simulink model "label_traj_calc"  (R2020b)
settings: Solver=FixedStepDiscrete  StartTime=0.0  StopTime=10.0  FixedStep=0.05  RelTol=1e-3
libraries: simulink x1
settings Model: Creator=chaoqun  LastModifiedBy=chaoqun
settings OptimizationCC: DefaultParameterBehavior=Inlined  EnhancedBackFolding=on  PassReuseOutputArgsAs=Individual arguments  ZeroExternalMemoryAtStartup=off  ZeroInternalMemoryAtStartup=off  OptimizeBlockOrder=speed  DifferentSizesBufferReuse=on  OptimizationCustomize=off  EfficientTunableParamExpr=on
settings DebuggingCC: ParameterTunabilityLossMsg=error
settings SFSimCC: MATLABDynamicMemAlloc=off
settings RTWCC: Description=Embedded Coder  SystemTargetFile=ert.tlc  GenCodeOnly=on  TemplateMakefile=ert_default_tmf
settings CodeAppCC: ForceParamTrailComments=on  IgnoreCustomStorageClasses=off  OperatorAnnotations=on  SimulinkDataObjDesc=on  SFDataObjDesc=on  InsertBlockDesc=on
settings ERTTargetCC: TargetLangStandard=C99 (ISO)  InlinedParameterPlacement=NonHierarchical  ERTCustomFileTemplate=example_file_process.tlc

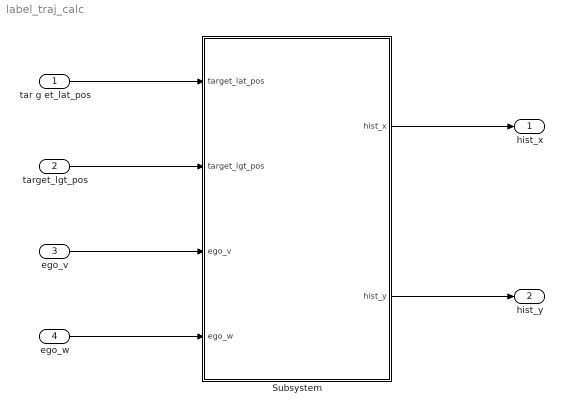
== system label_traj_calc ==
  tar g et_lat_pos : Inport  PortDimensions=100
  target_lgt_pos : Inport  Port=2  PortDimensions=100
  ego_v : Inport  Port=3  PortDimensions=100
  ego_w : Inport  Port=4  PortDimensions=100
  Subsystem : Subsystem
  hist_x : Outport
  hist_y : Outport  Port=2
  wires:
  tar g et_lat_pos/1 -> Subsystem/1(target_lat_pos)
  target_lgt_pos/1 -> Subsystem/2(target_lgt_pos)
  ego_v/1 -> Subsystem/3(ego_v)
  ego_w/1 -> Subsystem/4(ego_w)
  Subsystem/1(hist_x) -> hist_x/1
  Subsystem/2(hist_y) -> hist_y/1

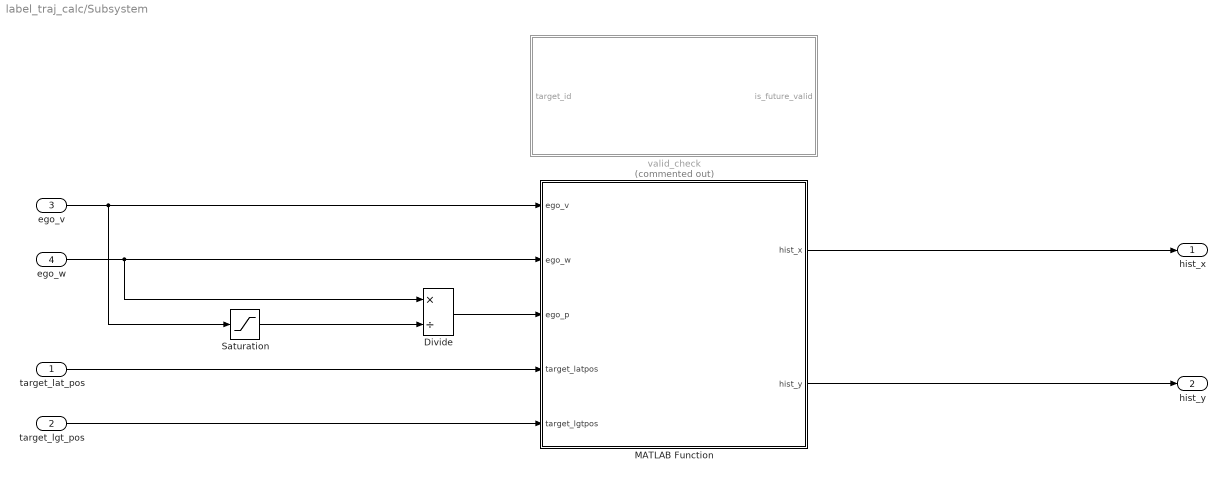
== system label_traj_calc/Subsystem ==
  target_lat_pos : Inport  PortDimensions=100
  target_lgt_pos : Inport  Port=2  PortDimensions=100
  ego_v : Inport  Port=3  PortDimensions=100
  ego_w : Inport  Port=4  PortDimensions=100
  Divide : Product  Inputs=*/
  MATLAB Function : MATLAB Function  TreatAsAtomicUnit=on
  Saturation : Saturate  UpperLimit=100  LowerLimit=1
  valid_check : Subsystem  Commented=on
  hist_x : Outport
  hist_y : Outport  Port=2
  wires:
  ego_w/1 -> MATLAB Function/2(ego_w), Divide/1
  Divide/1 -> MATLAB Function/3(ego_p)
  target_lat_pos/1 -> MATLAB Function/4(target_latpos)
  target_lgt_pos/1 -> MATLAB Function/5(target_lgtpos)
  MATLAB Function/2(hist_y) -> hist_y/1
  Saturation/1 -> Divide/2
  ego_v/1 -> MATLAB Function/1(ego_v), Saturation/1
  MATLAB Function/1(hist_x) -> hist_x/1

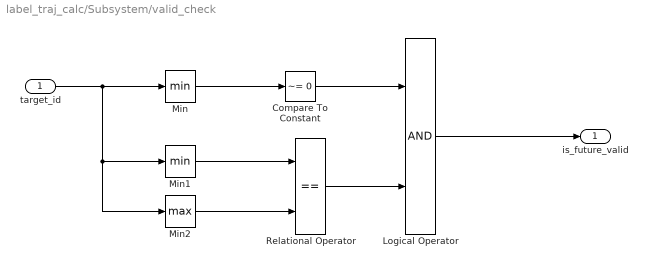
== system label_traj_calc/Subsystem/valid_check ==
  target_id : Inport
  Compare To Constant : simulink/Logic and Bit Operations/Compare To Constant  relop=~=  const=0  OutDataTypeStr=boolean
  Logical Operator : Logic  AllPortsSameDT=off  OutDataTypeStr=boolean
  Min : MinMax
  Min1 : MinMax
  Min2 : MinMax  Function=max
  Relational Operator : RelationalOperator  Operator===  OutDataTypeStr=boolean  RndMeth=Simplest
  is_future_valid : Outport
  wires:
  target_id/1 -> Min2/1, Min1/1, Min/1
  Min/1 -> Compare To Constant/1
  Compare To Constant/1 -> Logical Operator/1
  Relational Operator/1 -> Logical Operator/2
  Min2/1 -> Relational Operator/2
  Min1/1 -> Relational Operator/1
  Logical Operator/1 -> is_future_valid/1

== matlab function label_traj_calc/Subsystem/MATLAB Function ==
  data: ego_v input; ego_w input; ego_p input; target_latpos input; target_lgtpos input; hist_x output; hist_y output
function [hist_x, hist_y] = fcn(ego_v, ego_w, ego_p, target_latpos, target_lgtpos)

    hist_x = zeros(1,100);
    hist_y = zeros(1,100);

    dt = 0.05;


    for i=1:1:100
        psi= ego_w(100-i+1)*dt;

        dX = ego_v(100-i+1)*dt;

        dY = 0.5*ego_p(100-i+1)*dX*dX;


        % assign new target(x,y)
        hist_x(1, 100-i+1) = target_lgtpos(100-i+1);
        hist_y(1, 100-i+1) = target_latpos(100-i+1);


        [hist_x, hist_y] = coords_translate(-1*psi, -1*dX, -1*dY, hist_x, hist_y);


    end


end




function [X_t, Y_t] =  coords_translate(psi, dX, dY, X, Y)
% /*
% Transform Matrix is as following:   Move (dX, dY)m, Then Rotate (Psi) rad
% 
%          [  cos(psi)  sin(psi)  -(dX*cos(psi) + dY*sin(psi)) ;
% T =      -sin(psi)  cos(psi)   (dX*sin(psi)  -  dY*cos(psi));
%                      0             0                                           1  ]
% 
% */


% X_t =    X*cos(psi) + Y*sin(psi) - (dX*cos(psi) + dY*sin(psi));
% 
% Y_t = -1*X*sin(psi) + Y*cos(psi) + (dX*sin(psi)  -  dY*cos(psi));

X_t =    X*cos(psi) + Y*sin(psi) - dX;

Y_t =    -1*X*sin(psi) + Y*cos(psi) - dY;

end
